simulink subsystem "Aging"  (R2022a)
settings: Solver=VariableStepAuto  StartTime=0.0  StopTime=10.0  RelTol=1e-3
undefined symbols (not defined in the file or in its folder): Cn
libraries: simulink x1
settings Model: Creator=mateu  LastModifiedBy=mateu

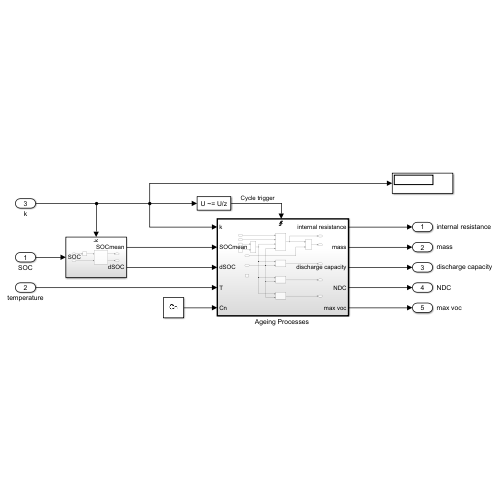
[thumbnail: Simulink's stored preview of the top-level diagram]
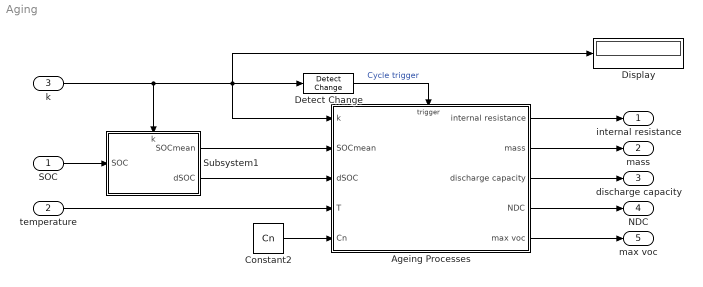
== system Aging ==
  SOC : Inport
  temperature : Inport  Port=2
  k : Inport  Port=3
  "Ageing Processes " : Subsystem
  Constant2 : Constant  Value=Cn
  Detect Change : simulink/Logic and Bit Operations/Detect Change  vinit=0  OutDataTypeStr=boolean
  Display : Display
  Subsystem1 : Subsystem
      settings: PortSchema="{\"entries\":[{\"content\":{\"sides\":[{\"content\":{\"connectorIds\":[\"In1\"]},\"type\":\"ConnectorPlacement.EquallySpacedRectSide\",\"uuid\":\"08511c64-fabd-454f-add4-1879c4ee32c0\"},{\"content\":{\"connectorIds\":[\"Out1\",\"Out2\"],\"side\":\"RIGHT\"},\"type\":\"ConnectorPlacement.EquallySpacedRectSide\",\"uuid\":\"e2e68503-dc42-4885-9f53-9ad148495dbe\"},{\"content\":{\"connectorIds\":[\"In2\"],\"side\":\"TOP\"},\"type\":\"ConnectorPlacement.EquallySpacedRectSide\",\"uuid\":\"dba375bd-a043-42fb-b865-3832d8025d62\"},{\"content\":{\"connectorIds\":[],\"side\":\"BOTTOM\"},\"type\":\"ConnectorPlacement.EquallySpacedRectSide\",\"uuid\":\"9b2cd940-abd2-4976-907f-d6152a0e047e\"}]},\"type\":\"ConnectorPlacement.EquallySpacedConnector\",\"uuid\":\"19562d64-d00a-4cef-b641-92a288dc47db\"}],\"packageUris\":[\"http://schema.mathworks.com/mf0/Connector/R2020b\"],\"version\":\"1.0\"}"
  internal resistance : Outport
  mass : Outport  Port=2
  discharge capacity : Outport  Port=3
  NDC : Outport  Port=4
  max voc : Outport  Port=5
  wires:
  "Ageing Processes "/3(discharge capacity) -> discharge capacity/1
  Subsystem1/2(dSOC) -> "Ageing Processes "/3(dSOC)
  "Ageing Processes "/4(NDC) -> NDC/1
  "Ageing Processes "/1(internal resistance) -> internal resistance/1
  "Ageing Processes "/2(mass) -> mass/1
  "Ageing Processes "/5(max voc) -> max voc/1
  Subsystem1/1(SOCmean) -> "Ageing Processes "/2(SOCmean)
  SOC/1 -> Subsystem1/1(SOC)
  temperature/1 -> "Ageing Processes "/4(T)
  Detect Change/1 -> "Ageing Processes "/Trigger  "Cycle trigger"
  Constant2/1 -> "Ageing Processes "/5(Cn)
  k/1 -> Display/1, "Ageing Processes "/1(k), Detect Change/1, Subsystem1/2(k)

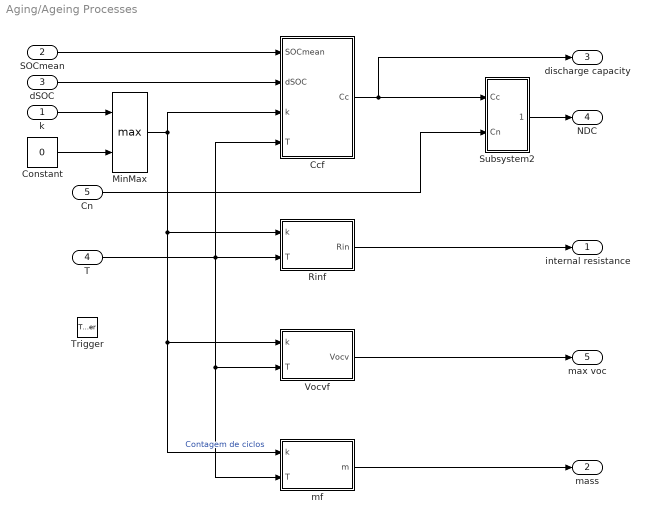
== system Aging/Ageing Processes  ==
  k : Inport
  SOCmean : Inport  Port=2
  dSOC : Inport  Port=3
  T : Inport  Port=4
  Cn : Inport  Port=5
  Trigger : TriggerPort  VariantControl=(inherit)  InitialTriggerSignalState=zero  PortDimensions=1
  Ccf : MATLAB Function  TreatAsAtomicUnit=on
  Constant : Constant  Value=0
  MinMax : MinMax  Function=max  Inputs=2
  Rinf : MATLAB Function  TreatAsAtomicUnit=on
  Subsystem2 : Subsystem
  Vocvf : MATLAB Function  TreatAsAtomicUnit=on
  mf : MATLAB Function  TreatAsAtomicUnit=on
  internal resistance : Outport
  mass : Outport  Port=2
  discharge capacity : Outport  Port=3
  NDC : Outport  Port=4
  max voc : Outport  Port=5
  wires:
  SOCmean/1 -> Ccf/1(SOCmean)
  MinMax/1 -> Rinf/1(k), Vocvf/1(k), mf/1(k), Ccf/3(k)  "Contagem de ciclos"
  dSOC/1 -> Ccf/2(dSOC)
  Rinf/1(Rin) -> internal resistance/1
  Subsystem2/1(NDC) -> NDC/1
  T/1 -> Rinf/2(T), Ccf/4(T), Vocvf/2(T), mf/2(T)
  Vocvf/1(Vocv) -> max voc/1
  Cn/1 -> Subsystem2/2(Cn)
  mf/1(m) -> mass/1
  Ccf/1(Cc) -> Subsystem2/1(Cc), discharge capacity/1
  k/1 -> MinMax/1
  Constant/1 -> MinMax/2

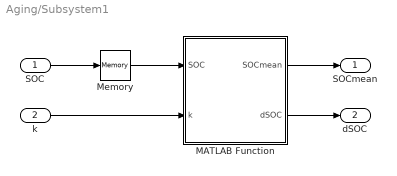
== system Aging/Subsystem1 ==
  SOC : Inport
  k : Inport  Port=2
  MATLAB Function : MATLAB Function  TreatAsAtomicUnit=on
  Memory : Memory  InheritSampleTime=on
  SOCmean : Outport
  dSOC : Outport  Port=2
  wires:
  k/1 -> MATLAB Function/2(k)
  Memory/1 -> MATLAB Function/1(SOC)
  MATLAB Function/1(SOCmean) -> SOCmean/1
  SOC/1 -> Memory/1
  MATLAB Function/2(dSOC) -> dSOC/1

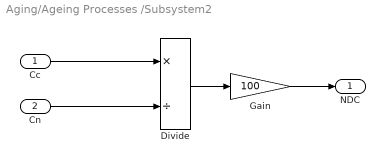
== system Aging/Ageing Processes /Subsystem2 ==
  Cc : Inport
  Cn : Inport  Port=2
  Divide : Product  Inputs=*/
  Gain : Gain  Gain=100
  NDC : Outport
  wires:
  Cc/1 -> Divide/1
  Gain/1 -> NDC/1
  Cn/1 -> Divide/2
  Divide/1 -> Gain/1

== matlab function Aging/Ageing Processes /Ccf ==
  data: SOCmean input; dSOC input; k input; Cc output; T input
function Cc = fcn(SOCmean, dSOC,k,T)
% Coeficients model Saxena2016
        k1 = 3.25;
        k2 = 3.25;
        k3 = -2.25;
% Coefficients (with 95% confidence bounds):
       p00 =       56.02;%  (53.93, 58.1)
       p10 =      -10.53;%  (-13.71, -7.36)
       p01 =       0.869;%  (-0.7052, 2.443)
       p20 =      -4.808;%  (-6.007, -3.609)
       p11 =      -1.445;%  (-2.534, -0.3554)
       p02 =      -1.223;%  (-2.763, 0.3179)
       p30 =      -2.931;%  (-4.53, -1.332)
       p21 =       -1.55;%  (-2.783, -0.3163)
       p12 =    -0.09181;%  (-1.677, 1.493)

       x = (k-9000)/6326;
       y = (T-31.67)/10.57;
       
%Linear model Poly32:
     fcn = p00 + p10*x + p01*y + p20*x^2 + p11*x*y + p02*y^2 + p30*x^3 + p21*x^2*y + p12*x*y^2;

     Cc = (100 - k1*SOCmean/100*(1+k2*dSOC/100+k3*(dSOC/100)^2) )/100*fcn;
                    
%       where x is normalized by mean 9000 and std 6326
%       and where y is normalized by mean 31.67 and std 10.57


% Goodness of fit:
%   SSE: 29.68
%   R-square: 0.9934
%   Adjusted R-square: 0.9875
%   RMSE: 1.816

== matlab function Aging/Ageing Processes /Rinf ==
  data: k input; Rin output; T input
function Rin = fcn(k,T)

       x = (k-9000)/6326;
       y = (T-31.67)/10.57;
       
%        where x is normalized by mean 9000 and std 6326
%        and where y is normalized by mean 31.67 and std 10.57
% Coefficients (with 95% confidence bounds):
       p00 =    0.003956;%  (0.003728, 0.004184)
       p10 =   0.0006753;%  (0.0004339, 0.0009166)
       p01 =  -1.804e-05;%  (-0.0001419, 0.0001059)
       p20 =   0.0005921;%  (0.000144, 0.00104)
       p11 =   0.0002673;%  (4.651e-05, 0.0004881)
       p02 =   3.119e-05;%  (-0.0001491, 0.0002115)
       p30 =   0.0001137;%  (-7.891e-06, 0.0002354)
       p21 =   0.0002022;%  (0.0001025, 0.0003019)
       p12 =  -0.0002286;%  (-0.0003492, -0.0001081)
       p40 =  -1.788e-05;%  (-0.0002076, 0.0001718)
       p31 =  -1.552e-05;%  (-0.0001407, 0.0001096)
       p22 =  -0.0001674;%  (-0.0003125, -2.232e-05)

       %Linear model Poly42:
     Rin = p00 + p10*x + p01*y + p20*x^2 + p11*x*y + p02*y^2 + p30*x^3 + p21*x^2*y ...
                    + p12*x*y^2 + p40*x^4 + p31*x^3*y + p22*x^2*y^2;

       
% Goodness of fit:
%   SSE: 9.784e-08
%   R-square: 0.991
%   Adjusted R-square: 0.9746
%   RMSE: 0.0001277

== matlab function Aging/Ageing Processes /Vocvf ==
  data: k input; Vocv output; T input
function Vocv = fcn(k,T)

%Coefficients (with 95% confidence bounds):
       p00 =       12.46;%  (12.4, 12.53)
       p10 =      0.2911;%  (0.2589, 0.3233)
       p01 =     0.03352;%  (-0.0006909, 0.06772)
       p20 =      0.0383;%  (-0.0004375, 0.07703)
       p11 =     0.02935;%  (-0.003774, 0.06248)
       p02 =    -0.01441;%  (-0.06418, 0.03537)

       x = (k-9000)/6326;
       y = (T-31.67)/10.57;
       
%Linear model Poly22:
     Vocv = p00 + p10*x + p01*y + p20*x^2 + p11*x*y + p02*y^2;
%       where x is normalized by mean 9000 and std 6326
%       and where y is normalized by mean 31.67 and std 10.57

%Goodness of fit:
%  SSE: 0.04454
%  R-square: 0.971
%  Adjusted R-square: 0.9588
%  RMSE: 0.06092

== matlab function Aging/Ageing Processes /mf ==
  data: k input; m output; T input
function m = fcn(k,T)

%Coefficients (with 95% confidence bounds):
       p00 =       19.64;%  (19.58, 19.69)
       p10 =     -0.5246;%  (-0.606, -0.4431)
       p01 =    -0.08727;%  (-0.1277, -0.04686)
       p20 =        0.06;%  (0.02923, 0.09077)
       p11 =    -0.04133;%  (-0.0693, -0.01337)
       p02 =    -0.04346;%  (-0.08301, -0.003916)
       p30 =     0.02928;%  (-0.01177, 0.07033)
       p21 =    -0.02198;%  (-0.05365, 0.009682)
       p12 =      0.0413;%  (0.0006076, 0.082)

       x = (k-9000)/6326;
       y = (T-31.67)/10.57;
       
% Linear model Poly32:
     m = p00 + p10*x + p01*y + p20*x^2 + p11*x*y + p02*y^2 + p30*x^3 + p21*x^2*y ...
                    + p12*x*y^2;
%        where x is normalized by mean 9000 and std 6326
%        and where y is normalized by mean 31.67 and std 10.57


% Goodness of fit:
%   SSE: 0.01956
%   R-square: 0.9946
%   Adjusted R-square: 0.9898
%   RMSE: 0.04662

== matlab function Aging/Subsystem1/MATLAB Function ==
  data: SOCmean output; SOC input; dSOC output; k input
function [SOCmean,dSOC] = fcn(SOC,k)
%% Main function
    persistent SOC_MIN SOC_MAX khold SOCmeanHold dSOCHold
    
    if isempty(SOC_MIN) || isempty(SOC_MAX) || isempty(khold) ...
            || isempty(SOCmeanHold) || isempty(dSOCHold)

        SOCmeanHold = 50;
        dSOCHold = 100;

        [SOC_MIN,SOC_MAX,khold] = reset(k);
    end
    
    if khold ~= k
        SOCmeanHold = (SOC_MAX + SOC_MIN)/2;
        dSOCHold = SOC_MAX - SOC_MIN;

        [SOC_MIN,SOC_MAX,khold] = reset(k);
    end
    
    SOC_MIN = min(SOC_MIN,SOC);
    SOC_MAX = max(SOC_MAX,SOC);

    SOCmean = SOCmeanHold;
    dSOC = dSOCHold;

%% Reset function
    function [SOC_MIN,SOC_MAX,khold] = reset(k)
        SOC_MIN = 100;
        SOC_MAX = 0;
        khold = k;
    end
end
